simulink model "vexarmcortex_BEST_IR_Sensor_LineFollower1"  (R2019a)
settings: Solver=FixedStepAuto  StartTime=0.0  StopTime=inf  RelTol=1e-3  EnableMultiTasking=on
libraries: vexarmcortexlib x3, vexcommonlib x1
settings Model: ExtModeTrigDuration=25  Creator=sseshadr  LastModifiedBy=josea
settings DataIOCC: ReturnWorkspaceOutputs=off
settings OptimizationCC: PassReuseOutputArgsAs=Individual arguments  MaxStackSize=64
settings DebuggingCC: ParameterTunabilityLossMsg=error  ArithmeticOperatorsInVariantConditions=warning
settings HardwareCC: ProdBitPerPointer=32  ProdBitPerSizeT=32  ProdBitPerPtrDiffT=32  ProdLargestAtomicInteger=Long  ProdLargestAtomicFloat=Double  ProdWordSize=32  ProdHWDeviceType=ARM Compatible->ARM Cortex
settings SFSimCC: SimUseLocalCustomCode=off  MATLABDynamicMemAlloc=off
settings RTWCC: SystemTargetFile=ert.tlc  HardwareBoard=ARM Cortex-based VEX Microcontroller  TLCOptions="-aInlineSetEventsForThisBaseRateFcn=TLC_FALSE -aSuppressMultiTaskScheduler=TLC_FALSE  -aRateBasedStepFcn=0"  TemplateMakefile=ert_default_tmf  GenerateReport=on  RTWUseLocalCustomCode=off  Toolchain=GNU Tools for VEX ARM Cortex  IncludeHyperlinkInReport=on  GenerateTraceInfo=on  GenerateTraceReport=on  GenerateTraceReportSl=on  GenerateTraceReportSf=on  GenerateTraceReportEml=on
settings CodeAppCC: ForceParamTrailComments=on  IgnoreCustomStorageClasses=off  OperatorAnnotations=on  SimulinkDataObjDesc=on  SFDataObjDesc=on  MATLABFcnDesc=on  InsertBlockDesc=on  StateflowObjectComments=on  MATLABSourceComments=on

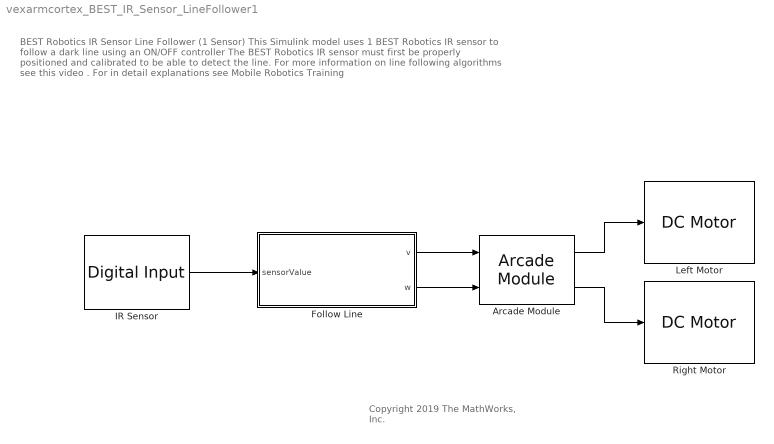
== system vexarmcortex_BEST_IR_Sensor_LineFollower1 ==
  note: BEST Robotics IR Sensor Line Follower (1 Sensor)
      |
      | This Simulink model uses 1 BEST Robotics IR sensor to follow a dark line using an ON/OFF controller
      | The BEST Robotics IR sensor must first be properly positioned and calibrated to be able to detect the line.
      | For more information on line following algorithms see this video .
      | For in detail explanations see Mobile Robotics Training
  note: Copyright 2019 The MathWorks, Inc.
  Arcade Module : vexcommonlib/Arcade Module  BlockPlatform=vexarmcortex
      settings: SourceProductName=Simulink Coder Support Package for ARM Cortex-based VEX Microcontroller  SourceProductBaseCode=EC_VEX_MICRO
  Follow Line : Stateflow chart  TreatAsAtomicUnit=on
  IR Sensor : vexarmcortexlib/Sensors/Digital Input  inChan=4  SimulationIn=off  SampleTime=0.05
      settings: SourceProductName=Simulink Coder Support Package for ARM Cortex-based VEX Microcontroller  SourceProductBaseCode=EC_VEX_MICRO
  Left Motor : vexarmcortexlib/Actuators/DC Motor  motor=5  scaleFactor=1/13.5  SimulationOut=off
      settings: SourceProductName=Simulink Coder Support Package for ARM Cortex-based VEX Microcontroller  SourceProductBaseCode=EC_VEX_MICRO
  Right Motor : vexarmcortexlib/Actuators/DC Motor  motor=3  scaleFactor=1/13.5  SimulationOut=off
      settings: SourceProductName=Simulink Coder Support Package for ARM Cortex-based VEX Microcontroller  SourceProductBaseCode=EC_VEX_MICRO
  wires:
  Arcade Module/2 -> Right Motor/1
  Arcade Module/1 -> Left Motor/1
  IR Sensor/1 -> Follow Line/1(sensorValue)
  Follow Line/2(w) -> Arcade Module/2
  Follow Line/1(v) -> Arcade Module/1

== stateflow chart vexarmcortex_BEST_IR_Sensor_LineFollower1/Follow Line ==
  state GoLeft
    entry:
    v = 50;
    w = 50;
  state GoRight
    entry:
    v = 50;
    w = -50;
  (default) -> GoLeft
  GoLeft -> GoRight : [sensorValue == 0]
  GoRight -> GoLeft : [sensorValue == 1]
  data: v output; w output; sensorValue input
